simulink model "drone_PD"  (Simulink 10.0)
settings: Solver=ode45  StartTime=0.0  StopTime=100  FixedStep=1e-3  RelTol=1e-5  EnableMultiTasking=on
values from neighbouring files (symbols this model uses):
  A = [0 0 1 0;0 0 0 1;0 0 -Kax/M 0;0 0 0 -Kay/M]    [modello_drone.m]
  B = [0 0;0 0;1/M 0;0 1/M]    [modello_drone.m]
  C = [1 0 0 0;0 1 0 0]    [modello_drone.m]
  D = zeros(2,5)    [modello_drone.m]
  G = [0 0 0 -1]'    [modello_drone.m]
  Mmax = 2,Mn=1.8    [modello_drone.m]
undefined symbols (not defined in the file or in its folder): Mn
libraries: simulink x1, simulink_need_slupdate x1
settings Model: Creator=prof. G. Celentano  LastModifiedBy=giuseppericcio
settings DataIOCC: LimitDataPoints=on  SignalLoggingSaveFormat=ModelDataLogs  SignalLoggingName=sigsOut
settings OptimizationCC: ExpressionDepthLimit=2147483647  InitFltsAndDblsToZero=on
settings DebuggingCC: SaveWithParameterizedLinksMsg=none  SignalResolutionControl=TryResolveAllWithWarning  MultiTaskDSMMsg=warning  MultiTaskCondExecSysMsg=none  FcnCallInpInsideContextMsg=warning  StateNameClashWarn=warning
settings HardwareCC: TargetUnknown=on
settings GRTTargetCC: TargetFcnLib=ansi_tfl_tmw.mat

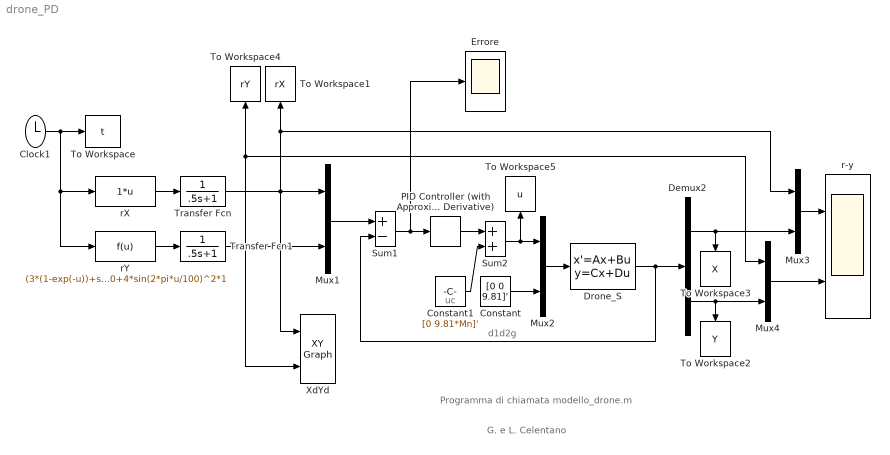
== system drone_PD ==
  note: G. e L. Celentano
  note: Programma di chiamata modello_drone.m
  note: d1d2g
  note: uc
  " Errore" : Scope
  " XdYd " : simulink/Sinks/XY Graph  xmin=0  xmax=100  ymin=0  ymax=5  st=-1
  Clock1 : Clock
  Constant : Constant  Value=[0 0 9.81]'
  Constant1 : Constant  Value=[0 9.81*Mn]'
  Demux2 : Demux  Outputs=2
  Drone_S : StateSpace  A=A  B=[B E G]  C=C  D=D  InitialCondition=0
  Mux1 : Mux  Inputs=[1 1]
  Mux2 : Mux  Inputs=[2 3]
  Mux3 : Mux  Inputs=[1 1]
  Mux4 : Mux  Inputs=[1 1]
  PID Controller (with Approximate Derivative) : simulink_need_slupdate/PID Controller (with Approximate Derivative)  P=Mmax*2*10^2  I=0  D=Mmax*2*10  N=100
      settings: SourceProductName=Simulink  SourceProductBaseCode=SL
  Sum1 : Sum  Inputs=+-  SaturateOnIntegerOverflow=on  InputSameDT=on  OutDataTypeStr=Inherit: Same as first input
  Sum2 : Sum  SaturateOnIntegerOverflow=on  InputSameDT=on  OutDataTypeStr=Inherit: Same as first input
  To Workspace : ToWorkspace  VariableName=t  SampleTime=-1
  To Workspace1 : ToWorkspace  VariableName=rX  SampleTime=-1
  To Workspace2 : ToWorkspace  VariableName=Y  SampleTime=-1
  To Workspace3 : ToWorkspace  VariableName=X  SampleTime=-1
  To Workspace4 : ToWorkspace  VariableName=rY  SampleTime=-1
  To Workspace5 : ToWorkspace  VariableName=u  SampleTime=-1
  Transfer Fcn : TransferFcn  Denominator=[.5 1]
  Transfer Fcn1 : TransferFcn  Denominator=[.5 1]
  r-y : Scope  NumInputPorts=2
  rX : Fcn  Expr=1*u
  rY : Fcn  Expr=(3*(1-exp(-u))+sin(2*pi/20*u))*0+4*sin(2*pi*u/100)^2*1
  wires:
  Drone_S/1 -> Demux2/1, Sum1/2
  Mux2/1 -> Drone_S/1
  Mux3/1 -> r-y/1
  Mux4/1 -> r-y/2
  Demux2/1 -> Mux3/2, To Workspace3/1
  Demux2/2 -> Mux4/2, To Workspace2/1
  Clock1/1 -> To Workspace/1, rX/1, rY/1
  Transfer Fcn/1 -> " XdYd "/1, To Workspace1/1, Mux3/1, Mux1/1
  rX/1 -> Transfer Fcn/1
  rY/1 -> Transfer Fcn1/1
  Transfer Fcn1/1 -> " XdYd "/2, To Workspace4/1, Mux4/1, Mux1/2
  Constant/1 -> Mux2/2
  Mux1/1 -> Sum1/1
  Sum1/1 -> PID Controller (with Approximate Derivative)/1, " Errore"/1
  Sum2/1 -> Mux2/1, To Workspace5/1
  PID Controller (with Approximate Derivative)/1 -> Sum2/1
  Constant1/1 -> Sum2/2
